simulink model "Four_Robots_v2"  (R2021a)
settings: Solver=FixedStepAuto  StartTime=0.0  StopTime=t_sim  FixedStep=0.01  RelTol=1e-3  EnableMultiTasking=on
model workspace (MAT data in the model file):
  SL_ROS_VariableLengthArrays_MaxSizes.CommonInfo.ArrayTruncateAction = 'EmitWarning'
  SL_ROS_VariableLengthArrays_MaxSizes.MsgTypeMap = containers.Map
  SL_ROS_VariableLengthArrays_MaxSizes.MsgTypeMap.serialization.keys = {'sensor_msgs/LaserScan'}
  SL_ROS_VariableLengthArrays_MaxSizes.MsgTypeMap.serialization.values{1}(1).PropertyName = 'Intensities'
  SL_ROS_VariableLengthArrays_MaxSizes.MsgTypeMap.serialization.values{1}(1).DataType = 'single'
  SL_ROS_VariableLengthArrays_MaxSizes.MsgTypeMap.serialization.values{1}(1).MaxLength = 360
  SL_ROS_VariableLengthArrays_MaxSizes.MsgTypeMap.serialization.values{1}(2).PropertyName = 'Ranges'
  SL_ROS_VariableLengthArrays_MaxSizes.MsgTypeMap.serialization.values{1}(2).DataType = 'single'
  SL_ROS_VariableLengthArrays_MaxSizes.MsgTypeMap.serialization.values{1}(2).MaxLength = 360
  SL_ROS_VariableLengthArrays_MaxSizes.MsgTypeMap.serialization.uniformity = 0
  SL_ROS_VariableLengthArrays_MaxSizes.MsgTypeMap.serialization.keyType = 'char'
  SL_ROS_VariableLengthArrays_MaxSizes.MsgTypeMap.serialization.valueType = 'any'
undefined symbols (not defined in the file or in its folder): Angular, Linear, PP, Way1, Way2, Way3, Way4
libraries: robotlib x16, robotalgslib x8
(part 1 of 2)
settings Model: EnablePacing=on  PacingRate=0.500000  Creator=The MathWorks, Inc.  LastModifiedBy=marco
settings SolverCC: AlgebraicLoopSolver=TrustRegion
settings DataIOCC: ReturnWorkspaceOutputs=off
settings OptimizationCC: EnhancedBackFolding=on  PassReuseOutputArgsAs=Individual arguments  ZeroExternalMemoryAtStartup=off  ZeroInternalMemoryAtStartup=off  MaxStackSize=64  OptimizeBlockOrder=speed  DifferentSizesBufferReuse=on  OptimizationCustomize=off  EfficientTunableParamExpr=on
settings DebuggingCC: ParameterTunabilityLossMsg=error  SFMachineParentedDataDiag=warning  ArithmeticOperatorsInVariantConditions=warning
settings HardwareCC: ProdBitPerPointer=32  ProdBitPerSizeT=32  ProdBitPerPtrDiffT=32  ProdLargestAtomicFloat=None  ProdIntDivRoundTo=Undefined  ProdEndianess=Unspecified  ProdWordSize=32  ProdHWDeviceType=Generic->Unspecified (assume 32-bit Generic)  UseEmbeddedCoderFeatures=off
settings SFSimCC: SimUseLocalCustomCode=off  MATLABDynamicMemAlloc=off  CustomCodeUndefinedFunction=UseInterfaceOnly
settings RTWCC: SystemTargetFile=ert.tlc  HardwareBoard=Robot Operating System (ROS)  TLCOptions="-aInlineSetEventsForThisBaseRateFcn=TLC_FALSE -aSuppressMultiTaskScheduler=TLC_FALSE  -aRateBasedStepFcn=0"  TemplateMakefile=ert_default_tmf  RTWUseLocalCustomCode=off  Toolchain=Catkin  TargetLang=C++
settings CodeAppCC: ForceParamTrailComments=on  IgnoreCustomStorageClasses=off  OperatorAnnotations=on  SimulinkDataObjDesc=on  SFDataObjDesc=on  InsertBlockDesc=on
settings ERTTargetCC: SupportNonInlinedSFcns=on
settings ConfigComp: CovMetricSettings=dsw  CovSaveCumulativeToWorkspaceVar=on  CovSaveSingleToWorkspaceVar=on  CovExternalEMLEnable=off

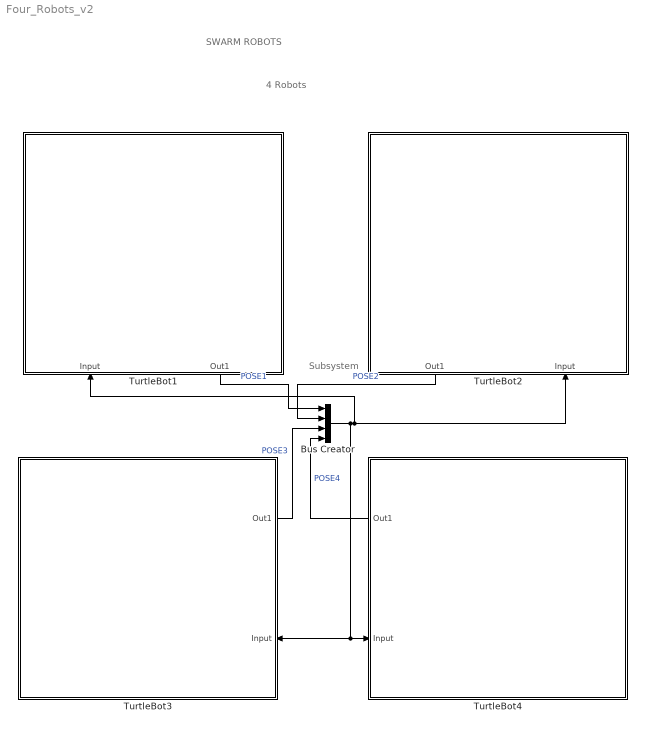
== system Four_Robots_v2 ==
  note: Subsystem
  note: SWARM ROBOTS
  note: 4 Robots
  Bus Creator : BusCreator  Inputs=4
  TurtleBot1 : Subsystem
      settings: PortSchema="{\"entries\":[{\"content\":{\"sides\":[{\"content\":{\"connectorIds\":[]},\"type\":\"ConnectorPlacement.EquallySpacedRectSide\",\"uuid\":\"56c3e334-5ee0-4d0f-bf2d-e3f55ae76ba4\"},{\"content\":{\"connectorIds\":[],\"side\":\"RIGHT\"},\"type\":\"ConnectorPlacement.EquallySpacedRectSide\",\"uuid\":\"47758117-cc89-48fb-b706-08d6cc9894c6\"},{\"content\":{\"connectorIds\":[],\"side\":\"TOP\"},\"type\":\"ConnectorPlacement.EquallySpacedRectSide\",\"uuid\":\"32d58290-5d9c-4684-a8aa-f76b0bdbcb35\"},{\"content\":{\"connectorIds\":[\"In1\",\"Out1\"],\"side\":\"BOTTOM\"},\"type\":\"ConnectorPlacement.EquallySpacedRectSide\",\"uuid\":\"a9083434-cc76-40d6-8718-10f7a0d9809f\"}]},\"type\":\"ConnectorPlacement.EquallySpacedConnector\",\"uuid\":\"5600436c-2c80-47b5-8769-67b5c2349f50\"}],\"packageUris\":[\"http://schema.mathworks.com/mf0/Connector/R2020b\"],\"version\":\"1.0\"}"
      mask Display: image('$imagefile'); % Use "Edit Image" on toolstrip to change.
  TurtleBot2 : Subsystem
      settings: PortSchema="{\"entries\":[{\"content\":{\"sides\":[{\"content\":{\"connectorIds\":[]},\"type\":\"ConnectorPlacement.EquallySpacedRectSide\",\"uuid\":\"56c3e334-5ee0-4d0f-bf2d-e3f55ae76ba4\"},{\"content\":{\"connectorIds\":[],\"side\":\"RIGHT\"},\"type\":\"ConnectorPlacement.EquallySpacedRectSide\",\"uuid\":\"47758117-cc89-48fb-b706-08d6cc9894c6\"},{\"content\":{\"connectorIds\":[],\"side\":\"TOP\"},\"type\":\"ConnectorPlacement.EquallySpacedRectSide\",\"uuid\":\"32d58290-5d9c-4684-a8aa-f76b0bdbcb35\"},{\"content\":{\"connectorIds\":[\"Out1\",\"In1\"],\"side\":\"BOTTOM\"},\"type\":\"ConnectorPlacement.EquallySpacedRectSide\",\"uuid\":\"a64cd998-99c6-4a68-9341-9505ecc52048\"}]},\"type\":\"ConnectorPlacement.EquallySpacedConnector\",\"uuid\":\"5600436c-2c80-47b5-8769-67b5c2349f50\"}],\"packageUris\":[\"http://schema.mathworks.com/mf0/Connector/R2020b\"],\"version\":\"1.0\"}"
      mask Display: image('$imagefile'); % Use "Edit Image" on toolstrip to change.
  TurtleBot3 : Subsystem
      settings: PortSchema="{\"entries\":[{\"content\":{\"sides\":[{\"content\":{\"connectorIds\":[]},\"type\":\"ConnectorPlacement.EquallySpacedRectSide\",\"uuid\":\"56c3e334-5ee0-4d0f-bf2d-e3f55ae76ba4\"},{\"content\":{\"connectorIds\":[\"Out1\",\"In1\"],\"side\":\"RIGHT\"},\"type\":\"ConnectorPlacement.EquallySpacedRectSide\",\"uuid\":\"47758117-cc89-48fb-b706-08d6cc9894c6\"},{\"content\":{\"connectorIds\":[],\"side\":\"TOP\"},\"type\":\"ConnectorPlacement.EquallySpacedRectSide\",\"uuid\":\"32d58290-5d9c-4684-a8aa-f76b0bdbcb35\"}]},\"type\":\"ConnectorPlacement.EquallySpacedConnector\",\"uuid\":\"5600436c-2c80-47b5-8769-67b5c2349f50\"}],\"packageUris\":[\"http://schema.mathworks.com/mf0/Connector/R2020b\"],\"version\":\"1.0\"}"
      mask Display: image('$imagefile'); % Use "Edit Image" on toolstrip to change.
  TurtleBot4 : Subsystem
      settings: PortSchema="{\"entries\":[{\"content\":{\"sides\":[{\"content\":{\"connectorIds\":[\"Out1\",\"In1\"]},\"type\":\"ConnectorPlacement.EquallySpacedRectSide\",\"uuid\":\"329d0968-fe7b-48af-96d4-efcc8444baaa\"},{\"content\":{\"connectorIds\":[],\"side\":\"RIGHT\"},\"type\":\"ConnectorPlacement.EquallySpacedRectSide\",\"uuid\":\"6b63acff-04c0-4cf0-89c5-b9cc2038ae37\"},{\"content\":{\"connectorIds\":[],\"side\":\"TOP\"},\"type\":\"ConnectorPlacement.EquallySpacedRectSide\",\"uuid\":\"86dad342-95f2-4c72-a91f-a7852aa38f6d\"}]},\"type\":\"ConnectorPlacement.EquallySpacedConnector\",\"uuid\":\"8a373283-c962-469e-9517-5e5763347250\"}],\"packageUris\":[\"http://schema.mathworks.com/mf0/Connector/R2020b\"],\"version\":\"1.0\"}"
      mask Display: image('$imagefile'); % Use "Edit Image" on toolstrip to change.
  wires:
  Bus Creator/1 -> TurtleBot4/1(Input), TurtleBot3/1(Input), TurtleBot1/1(Input), TurtleBot2/1(Input)
  TurtleBot3/1(Out1) -> Bus Creator/3  "POSE3"
  TurtleBot2/1(Out1) -> Bus Creator/2  "POSE2"
  TurtleBot4/1(Out1) -> Bus Creator/4  "POSE4"
  TurtleBot1/1(Out1) -> Bus Creator/1  "POSE1"

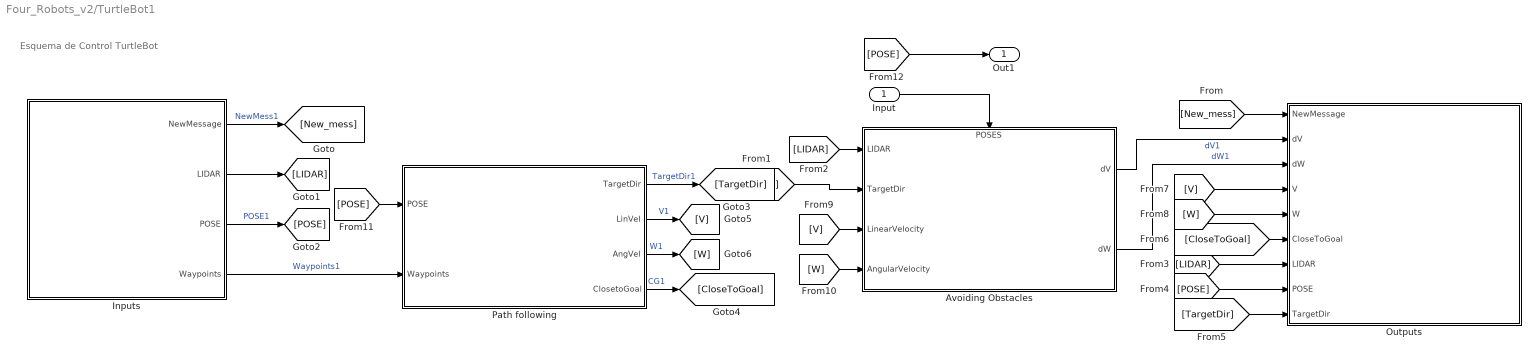
== system Four_Robots_v2/TurtleBot1 ==
  note: Esquema de Control TurtleBot
  Input : Inport
  " Avoiding Obstacles" : Subsystem
      settings: PortSchema="{\"entries\":[{\"content\":{\"sides\":[{\"content\":{\"connectorIds\":[\"In1\",\"In2\",\"In3\",\"In4\"]},\"type\":\"ConnectorPlacement.EquallySpacedRectSide\",\"uuid\":\"727160c1-1339-4bf3-a065-3e6cd81c52df\"},{\"content\":{\"connectorIds\":[\"Out1\",\"Out2\"],\"side\":\"RIGHT\"},\"type\":\"ConnectorPlacement.EquallySpacedRectSide\",\"uuid\":\"5e522eed-56ec-44ed-85e8-de700c46da17\"},{\"content\":{\"connectorIds\":[\"In5\"],\"side\":\"TOP\"},\"type\":\"ConnectorPlacement.EquallySpacedRectSide\",\"uuid\":\"c128634c-8085-427a-ae3a-e5a428db6a0b\"}]},\"type\":\"ConnectorPlacement.EquallySpacedConnector\",\"uuid\":\"85c8e4f2-74e0-4ae3-8945-7ca4be034673\"}],\"packageUris\":[\"http://schema.mathworks.com/mf0/Connector/R2020b\"],\"version\":\"1.0\"}"
      mask Display: image('$imagefile'); % Use "Edit Image" on toolstrip to change.
  " Path following" : Subsystem
      mask Display: image('$imagefile'); % Use "Edit Image" on toolstrip to change.
  Inputs : Subsystem
      mask Display: image('$imagefile'); % Use "Edit Image" on toolstrip to change.
  Outputs : Subsystem
      mask Display: image('$imagefile'); % Use "Edit Image" on toolstrip to change.
  Out1 : Outport
  wires:
  Inputs/3(POSE) -> [POSE]  "POSE1"
  Inputs/1(NewMessage) -> [New_mess]  "NewMess1"
  Inputs/2(LIDAR) -> [LIDAR]
  Inputs/4(Waypoints) -> " Path following"/2(Waypoints)  "Waypoints1"
  " Path following"/4(ClosetoGoal) -> [CloseToGoal]  "CG1"
  [LIDAR] -> " Avoiding Obstacles"/1(LIDAR)
  [New_mess] -> Outputs/1(NewMessage)
  [V] -> Outputs/4(V)
  [W] -> Outputs/5(W)
  [CloseToGoal] -> Outputs/6(CloseToGoal)
  [LIDAR] -> Outputs/7(LIDAR)
  [POSE] -> Outputs/8(POSE)
  [TargetDir] -> Outputs/9(TargetDir)
  " Path following"/1(TargetDir) -> [TargetDir]  "TargetDir1"
  " Avoiding Obstacles"/1(dV) -> Outputs/2(dV)  "dV1"
  " Avoiding Obstacles"/2(dW) -> Outputs/3(dW)  "dW1"
  " Path following"/3(AngVel) -> [W]  "W1"
  " Path following"/2(LinVel) -> [V]  "V1"
  [TargetDir] -> " Avoiding Obstacles"/2(TargetDir)
  [V] -> " Avoiding Obstacles"/3(LinearVelocity)
  [W] -> " Avoiding Obstacles"/4(AngularVelocity)
  [POSE] -> " Path following"/1(POSE)
  [POSE] -> Out1/1
  Input/1 -> " Avoiding Obstacles"/5(POSES)

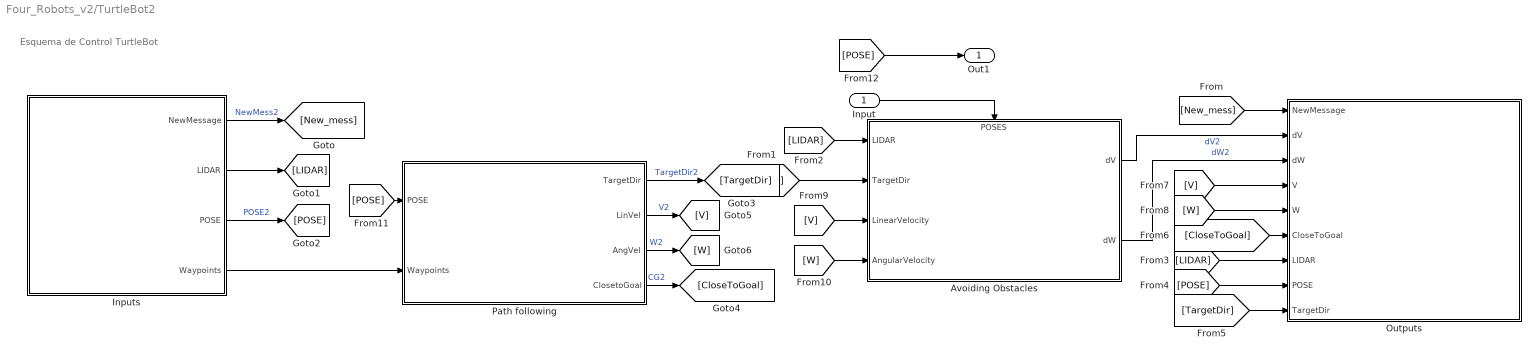
== system Four_Robots_v2/TurtleBot2 ==
  note: Esquema de Control TurtleBot
  Input : Inport
  " Avoiding Obstacles" : Subsystem
      settings: PortSchema="{\"entries\":[{\"content\":{\"sides\":[{\"content\":{\"connectorIds\":[\"In1\",\"In2\",\"In3\",\"In4\"]},\"type\":\"ConnectorPlacement.EquallySpacedRectSide\",\"uuid\":\"727160c1-1339-4bf3-a065-3e6cd81c52df\"},{\"content\":{\"connectorIds\":[\"Out1\",\"Out2\"],\"side\":\"RIGHT\"},\"type\":\"ConnectorPlacement.EquallySpacedRectSide\",\"uuid\":\"5e522eed-56ec-44ed-85e8-de700c46da17\"},{\"content\":{\"connectorIds\":[\"In5\"],\"side\":\"TOP\"},\"type\":\"ConnectorPlacement.EquallySpacedRectSide\",\"uuid\":\"c128634c-8085-427a-ae3a-e5a428db6a0b\"}]},\"type\":\"ConnectorPlacement.EquallySpacedConnector\",\"uuid\":\"85c8e4f2-74e0-4ae3-8945-7ca4be034673\"}],\"packageUris\":[\"http://schema.mathworks.com/mf0/Connector/R2020b\"],\"version\":\"1.0\"}"
      mask Display: image('$imagefile'); % Use "Edit Image" on toolstrip to change.
  " Path following" : Subsystem
      mask Display: image('$imagefile'); % Use "Edit Image" on toolstrip to change.
  Inputs : Subsystem
      mask Display: image('$imagefile'); % Use "Edit Image" on toolstrip to change.
  Outputs : Subsystem
      mask Display: image('$imagefile'); % Use "Edit Image" on toolstrip to change.
  Out1 : Outport
  wires:
  Inputs/3(POSE) -> [POSE]  "POSE2"
  Inputs/1(NewMessage) -> [New_mess]  "NewMess2"
  Inputs/2(LIDAR) -> [LIDAR]
  Inputs/4(Waypoints) -> " Path following"/2(Waypoints)
  " Path following"/4(ClosetoGoal) -> [CloseToGoal]  "CG2"
  [LIDAR] -> " Avoiding Obstacles"/1(LIDAR)
  [New_mess] -> Outputs/1(NewMessage)
  [V] -> Outputs/4(V)
  [W] -> Outputs/5(W)
  [CloseToGoal] -> Outputs/6(CloseToGoal)
  [LIDAR] -> Outputs/7(LIDAR)
  [POSE] -> Outputs/8(POSE)
  [TargetDir] -> Outputs/9(TargetDir)
  " Path following"/1(TargetDir) -> [TargetDir]  "TargetDir2"
  " Avoiding Obstacles"/1(dV) -> Outputs/2(dV)  "dV2"
  " Avoiding Obstacles"/2(dW) -> Outputs/3(dW)  "dW2"
  " Path following"/3(AngVel) -> [W]  "W2"
  " Path following"/2(LinVel) -> [V]  "V2"
  [TargetDir] -> " Avoiding Obstacles"/2(TargetDir)
  [V] -> " Avoiding Obstacles"/3(LinearVelocity)
  [W] -> " Avoiding Obstacles"/4(AngularVelocity)
  [POSE] -> " Path following"/1(POSE)
  Input/1 -> " Avoiding Obstacles"/5(POSES)
  [POSE] -> Out1/1

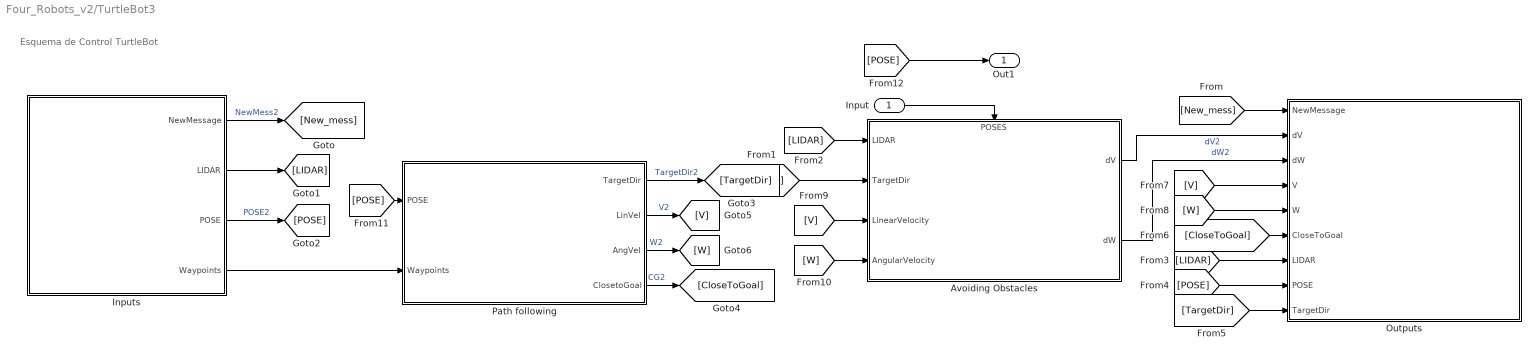
== system Four_Robots_v2/TurtleBot3 ==
  note: Esquema de Control TurtleBot
  Input : Inport
  " Avoiding Obstacles" : Subsystem
      settings: PortSchema="{\"entries\":[{\"content\":{\"sides\":[{\"content\":{\"connectorIds\":[\"In1\",\"In2\",\"In3\",\"In4\"]},\"type\":\"ConnectorPlacement.EquallySpacedRectSide\",\"uuid\":\"727160c1-1339-4bf3-a065-3e6cd81c52df\"},{\"content\":{\"connectorIds\":[\"Out1\",\"Out2\"],\"side\":\"RIGHT\"},\"type\":\"ConnectorPlacement.EquallySpacedRectSide\",\"uuid\":\"5e522eed-56ec-44ed-85e8-de700c46da17\"},{\"content\":{\"connectorIds\":[\"In5\"],\"side\":\"TOP\"},\"type\":\"ConnectorPlacement.EquallySpacedRectSide\",\"uuid\":\"c128634c-8085-427a-ae3a-e5a428db6a0b\"}]},\"type\":\"ConnectorPlacement.EquallySpacedConnector\",\"uuid\":\"85c8e4f2-74e0-4ae3-8945-7ca4be034673\"}],\"packageUris\":[\"http://schema.mathworks.com/mf0/Connector/R2020b\"],\"version\":\"1.0\"}"
      mask Display: image('$imagefile'); % Use "Edit Image" on toolstrip to change.
  " Path following" : Subsystem
      mask Display: image('$imagefile'); % Use "Edit Image" on toolstrip to change.
  Inputs : Subsystem
      mask Display: image('$imagefile'); % Use "Edit Image" on toolstrip to change.
  Outputs : Subsystem
      mask Display: image('$imagefile'); % Use "Edit Image" on toolstrip to change.
  Out1 : Outport
  wires:
  Inputs/3(POSE) -> [POSE]  "POSE2"
  Inputs/1(NewMessage) -> [New_mess]  "NewMess2"
  Inputs/2(LIDAR) -> [LIDAR]
  Inputs/4(Waypoints) -> " Path following"/2(Waypoints)
  " Path following"/4(ClosetoGoal) -> [CloseToGoal]  "CG2"
  [LIDAR] -> " Avoiding Obstacles"/1(LIDAR)
  [New_mess] -> Outputs/1(NewMessage)
  [V] -> Outputs/4(V)
  [W] -> Outputs/5(W)
  [CloseToGoal] -> Outputs/6(CloseToGoal)
  [LIDAR] -> Outputs/7(LIDAR)
  [POSE] -> Outputs/8(POSE)
  [TargetDir] -> Outputs/9(TargetDir)
  " Path following"/1(TargetDir) -> [TargetDir]  "TargetDir2"
  " Avoiding Obstacles"/1(dV) -> Outputs/2(dV)  "dV2"
  " Avoiding Obstacles"/2(dW) -> Outputs/3(dW)  "dW2"
  " Path following"/3(AngVel) -> [W]  "W2"
  " Path following"/2(LinVel) -> [V]  "V2"
  [TargetDir] -> " Avoiding Obstacles"/2(TargetDir)
  [V] -> " Avoiding Obstacles"/3(LinearVelocity)
  [W] -> " Avoiding Obstacles"/4(AngularVelocity)
  [POSE] -> " Path following"/1(POSE)
  [POSE] -> Out1/1
  Input/1 -> " Avoiding Obstacles"/5(POSES)

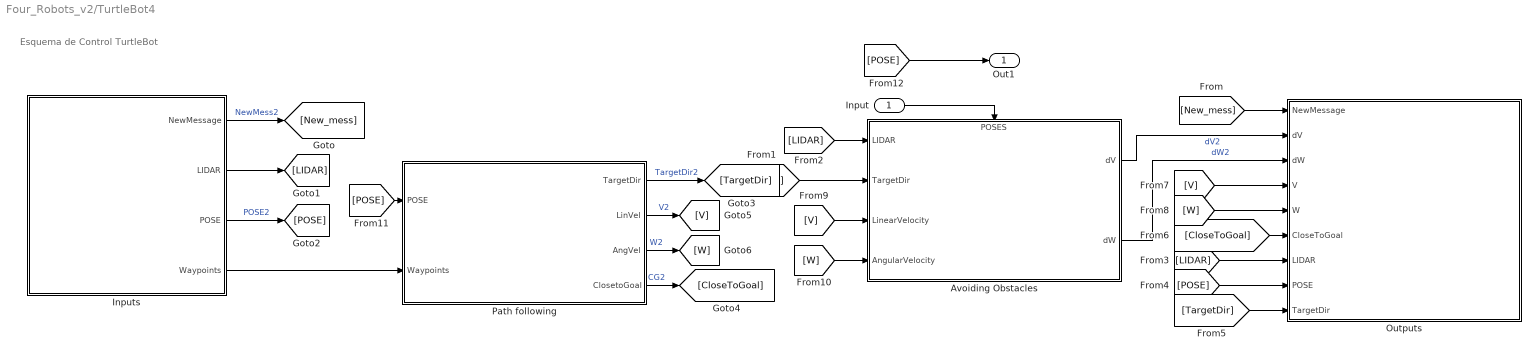
== system Four_Robots_v2/TurtleBot4 ==
  note: Esquema de Control TurtleBot
  Input : Inport
  " Avoiding Obstacles" : Subsystem
      settings: PortSchema="{\"entries\":[{\"content\":{\"sides\":[{\"content\":{\"connectorIds\":[\"In1\",\"In2\",\"In3\",\"In4\"]},\"type\":\"ConnectorPlacement.EquallySpacedRectSide\",\"uuid\":\"727160c1-1339-4bf3-a065-3e6cd81c52df\"},{\"content\":{\"connectorIds\":[\"Out1\",\"Out2\"],\"side\":\"RIGHT\"},\"type\":\"ConnectorPlacement.EquallySpacedRectSide\",\"uuid\":\"5e522eed-56ec-44ed-85e8-de700c46da17\"},{\"content\":{\"connectorIds\":[\"In5\"],\"side\":\"TOP\"},\"type\":\"ConnectorPlacement.EquallySpacedRectSide\",\"uuid\":\"c128634c-8085-427a-ae3a-e5a428db6a0b\"}]},\"type\":\"ConnectorPlacement.EquallySpacedConnector\",\"uuid\":\"85c8e4f2-74e0-4ae3-8945-7ca4be034673\"}],\"packageUris\":[\"http://schema.mathworks.com/mf0/Connector/R2020b\"],\"version\":\"1.0\"}"
      mask Display: image('$imagefile'); % Use "Edit Image" on toolstrip to change.
  " Path following" : Subsystem
      mask Display: image('$imagefile'); % Use "Edit Image" on toolstrip to change.
  Inputs : Subsystem
      mask Display: image('$imagefile'); % Use "Edit Image" on toolstrip to change.
  Outputs : Subsystem
      mask Display: image('$imagefile'); % Use "Edit Image" on toolstrip to change.
  Out1 : Outport
  wires:
  Input/1 -> " Avoiding Obstacles"/5(POSES)
  [POSE] -> Out1/1
  [POSE] -> " Path following"/1(POSE)
  [W] -> " Avoiding Obstacles"/4(AngularVelocity)
  [V] -> " Avoiding Obstacles"/3(LinearVelocity)
  [TargetDir] -> " Avoiding Obstacles"/2(TargetDir)
  " Path following"/2(LinVel) -> [V]  "V2"
  " Path following"/3(AngVel) -> [W]  "W2"
  " Avoiding Obstacles"/2(dW) -> Outputs/3(dW)  "dW2"
  " Avoiding Obstacles"/1(dV) -> Outputs/2(dV)  "dV2"
  " Path following"/1(TargetDir) -> [TargetDir]  "TargetDir2"
  [TargetDir] -> Outputs/9(TargetDir)
  [POSE] -> Outputs/8(POSE)
  [LIDAR] -> Outputs/7(LIDAR)
  [CloseToGoal] -> Outputs/6(CloseToGoal)
  [W] -> Outputs/5(W)
  [V] -> Outputs/4(V)
  [New_mess] -> Outputs/1(NewMessage)
  [LIDAR] -> " Avoiding Obstacles"/1(LIDAR)
  " Path following"/4(ClosetoGoal) -> [CloseToGoal]  "CG2"
  Inputs/4(Waypoints) -> " Path following"/2(Waypoints)
  Inputs/2(LIDAR) -> [LIDAR]
  Inputs/1(NewMessage) -> [New_mess]  "NewMess2"
  Inputs/3(POSE) -> [POSE]  "POSE2"

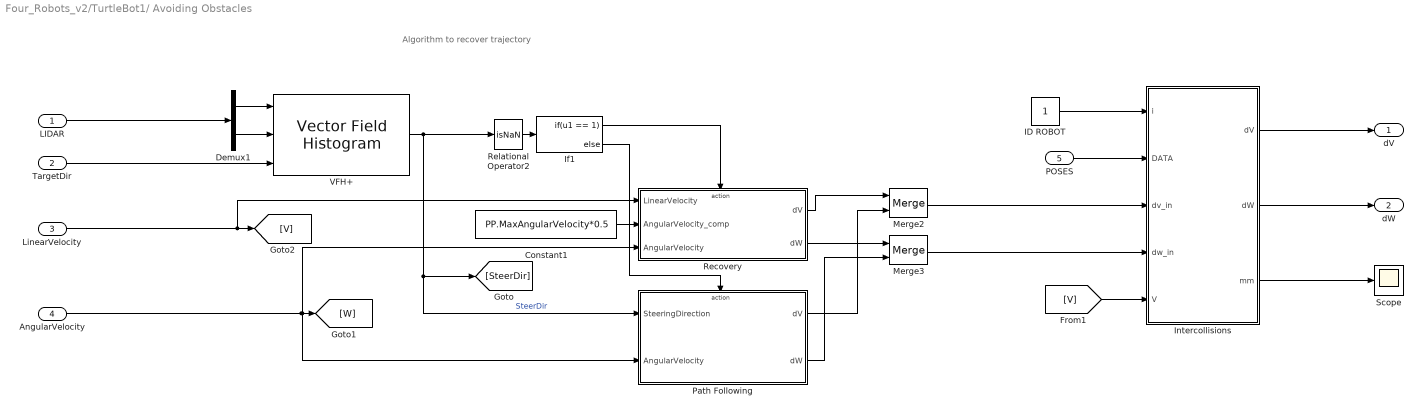
== system Four_Robots_v2/TurtleBot1/ Avoiding Obstacles ==
  note: Algorithm to recover trajectory
  LIDAR : Inport
  TargetDir : Inport  Port=2
  LinearVelocity : Inport  Port=3
  AngularVelocity : Inport  Port=4
  POSES : Inport  Port=5
  Constant1 : Constant  Value=PP.MaxAngularVelocity*0.5
  Demux1 : Demux  Outputs=2
  ID ROBOT : Constant
  If1 : If  IfExpression=u1 == 1
  Intercollisions : MATLAB Function  TreatAsAtomicUnit=on
  Merge2 : Merge
  Merge3 : Merge
  Path Following : Subsystem  TreatAsAtomicUnit=on
  Recovery : Subsystem  TreatAsAtomicUnit=on
  Relational Operator2 : RelationalOperator  Operator=isNaN  OutDataTypeStr=boolean  RndMeth=Simplest
  Scope : Scope
  VFH+ : robotalgslib/Vector Field Histogram  NumAngularSectors=VFH.NumAngularSectors  DistanceLimits=VFH.DistanceLimits  HistogramThresholds=VFH.HistogramThresholds  RobotRadius=VFH.RobotRadius  SafetyDistance=VFH.SafetyDistance  MinTurningRadius=VFH.MinTurningRadius  SimulateUsing=Code generation  TargetDirectionWeight=5  CurrentDirectionWeight=2  PreviousDirectionWeight=2
      settings: SourceProductBaseCode=NV,RO
  dV : Outport
  dW : Outport  Port=2
  wires:
  If1/1 -> Recovery/Action
  Constant1/1 -> Recovery/2(AngularVelocity_comp)
  Recovery/1(dV) -> Merge2/1
  Recovery/2(dW) -> Merge3/1
  AngularVelocity/1 -> Recovery/3(AngularVelocity), Path Following/2(AngularVelocity), [W]
  Demux1/1 -> VFH+/1
  TargetDir/1 -> VFH+/3
  Relational Operator2/1 -> If1/1
  LinearVelocity/1 -> [V], Recovery/1(LinearVelocity)
  LIDAR/1 -> Demux1/1
  VFH+/1 -> [SteerDir], Path Following/1(SteeringDirection), Relational Operator2/1  "SteerDir"
  Path Following/2(dW) -> Merge3/2
  Path Following/1(dV) -> Merge2/2
  If1/2 -> Path Following/Action
  Demux1/2 -> VFH+/2
  Intercollisions/2(dW) -> dW/1
  [V] -> Intercollisions/5(V)
  Merge2/1 -> Intercollisions/3(dv_in)
  Merge3/1 -> Intercollisions/4(dw_in)
  Intercollisions/1(dV) -> dV/1
  ID ROBOT/1 -> Intercollisions/1(i)
  POSES/1 -> Intercollisions/2(DATA)
  Intercollisions/3(mm) -> Scope/1

== system Four_Robots_v2/TurtleBot1/ Path following ==
  note: Check If Close To Goal
  POSE : Inport
  Waypoints : Inport  Port=2
  " Extract Goal" : MATLAB Function  TreatAsAtomicUnit=on
  Dot Product : DotProduct  InputSameDT=on  OutDataTypeStr=Inherit: Inherit via internal rule
  GoalRadius : Constant  Value=0.15
  Pure Pursuit : robotalgslib/Pure Pursuit  DesiredLinearVelocity=PP.DesiredLinearVelocity  MaxAngularVelocity=PP.MaxAngularVelocity  LookaheadDistance=PP.LookaheadDistance  TargetDirPort=on  SimulateUsing=Code generation
  Relational Operator : RelationalOperator  Operator=<=  OutDataTypeStr=boolean  RndMeth=Simplest
  Selector : Selector  InputPortWidth=3  IndexOptions=Index vector (dialog)  Indices=[1 2]  OutputSizes=1
  Sqrt : Sqrt  SaturateOnIntegerOverflow=on
  Subtract : Sum  Inputs=|+-
  TargetDir : Outport
  LinVel : Outport  Port=2
  AngVel : Outport  Port=3
  ClosetoGoal : Outport  Port=4
  wires:
  Pure Pursuit/3 -> TargetDir/1
  Pure Pursuit/2 -> AngVel/1
  Relational Operator/1 -> ClosetoGoal/1
  Subtract/1 -> Dot Product/1, Dot Product/2
  " Extract Goal"/1(Goal) -> Subtract/2
  Dot Product/1 -> Sqrt/1
  Pure Pursuit/1 -> LinVel/1
  Selector/1 -> Subtract/1
  Waypoints/1 -> " Extract Goal"/1(Waypoints), Pure Pursuit/2
  Sqrt/1 -> Relational Operator/1
  GoalRadius/1 -> Relational Operator/2
  POSE/1 -> Selector/1, Pure Pursuit/1

== system Four_Robots_v2/TurtleBot1/Inputs ==
  note: Receive Laser Message
  note: Receive Robot Pose
  Bus Selector : BusSelector  OutputSignals=Pose.Pose.Position.X,Pose.Pose.Position.Y,Pose.Pose.Orientation.X,Pose.Pose.Orientation.Y,Pose.Pose.Orientation.Z,Pose.Pose.Orientation.W
  MATLAB Function : MATLAB Function  TreatAsAtomicUnit=on
  Mux : Mux  Inputs=3
  Mux1 : Mux  Inputs=2
  Subscribe : robotlib/Subscribe  topicSource=Select from ROS network  topic=/robot1/scan  messageType=sensor_msgs/LaserScan  SampleTime=-1  legacyBusStruct=off  messageQueueLength=1
  Subscribe1 : robotlib/Subscribe  topicSource=Select from ROS network  topic=/robot1/odom  messageType=nav_msgs/Odometry  SampleTime=-1  legacyBusStruct=off  messageQueueLength=1
  Terminator : Terminator
  Waypoints Input1 : Constant  Value=Way1  OutDataTypeStr=double
  quad2eul : MATLAB Function  TreatAsAtomicUnit=on
  NewMessage : Outport
  LIDAR : Outport  Port=2
  POSE : Outport  Port=3
  Waypoints : Outport  Port=4
  wires:
  Bus Selector/6 -> quad2eul/4(W)  "<W>"
  Bus Selector/1 -> Mux/1  "<X>"
  quad2eul/1(Yaw) -> Mux/3
  Bus Selector/4 -> quad2eul/2(Y)  "<Y>"
  Subscribe1/2 -> Bus Selector/1
  MATLAB Function/1(Ranges) -> Mux1/1
  Mux/1 -> POSE/1
  Subscribe/2 -> MATLAB Function/1(LaserScanMsg)
  Subscribe/1 -> NewMessage/1
  Subscribe1/1 -> Terminator/1
  Bus Selector/3 -> quad2eul/1(X)  "<X>"
  Bus Selector/2 -> Mux/2  "<Y>"
  MATLAB Function/2(Angles) -> Mux1/2
  Mux1/1 -> LIDAR/1
  Waypoints Input1/1 -> Waypoints/1
  Bus Selector/5 -> quad2eul/3(Z)  "<Z>"

== system Four_Robots_v2/TurtleBot1/Outputs ==
  NewMessage : Inport
  dV : Inport  Port=2
  dW : Inport  Port=3
  V : Inport  Port=4
  W : Inport  Port=5
  CloseToGoal : Inport  Port=6
  LIDAR : Inport  Port=7
  POSE : Inport  Port=8
  TargetDir : Inport  Port=9
  DVelocities : Scope  NumInputPorts=2
  Outputs : Subsystem
  wires:
  POSE/1 -> Outputs/7(POSE)
  V/1 -> Outputs/3(V)
  NewMessage/1 -> Outputs/Enable
  CloseToGoal/1 -> Outputs/5(CloseToGoal)
  LIDAR/1 -> Outputs/6(LIDAR)
  TargetDir/1 -> Outputs/8(TargetDir)
  W/1 -> Outputs/4(W)
  dV/1 -> DVelocities/1, Outputs/1(dV)
  dW/1 -> DVelocities/2, Outputs/2(dW)

== system Four_Robots_v2/TurtleBot2/ Avoiding Obstacles ==
  note: Algorithm to recover trajectory
  LIDAR : Inport
  TargetDir : Inport  Port=2
  LinearVelocity : Inport  Port=3
  AngularVelocity : Inport  Port=4
  POSES : Inport  Port=5
  Constant1 : Constant  Value=PP.MaxAngularVelocity*0.5
  Demux1 : Demux  Outputs=2
  ID ROBOT : Constant  Value=2
  If1 : If  IfExpression=u1 == 1
  Intercollisions : MATLAB Function  TreatAsAtomicUnit=on
  Merge2 : Merge
  Merge3 : Merge
  Path Following : Subsystem  TreatAsAtomicUnit=on
  Recovery : Subsystem  TreatAsAtomicUnit=on
  Relational Operator2 : RelationalOperator  Operator=isNaN  OutDataTypeStr=boolean  RndMeth=Simplest
  VFH+ : robotalgslib/Vector Field Histogram  NumAngularSectors=VFH.NumAngularSectors  DistanceLimits=VFH.DistanceLimits  HistogramThresholds=VFH.HistogramThresholds  RobotRadius=VFH.RobotRadius  SafetyDistance=VFH.SafetyDistance  MinTurningRadius=VFH.MinTurningRadius  SimulateUsing=Code generation  TargetDirectionWeight=5  CurrentDirectionWeight=2  PreviousDirectionWeight=2
      settings: SourceProductBaseCode=NV,RO
  dV : Outport
  dW : Outport  Port=2
  wires:
  If1/1 -> Recovery/Action
  Constant1/1 -> Recovery/2(AngularVelocity_comp)
  Recovery/1(dV) -> Merge2/1
  Recovery/2(dW) -> Merge3/1
  AngularVelocity/1 -> Recovery/3(AngularVelocity), Path Following/2(AngularVelocity), [W]
  Demux1/1 -> VFH+/1
  TargetDir/1 -> VFH+/3
  Relational Operator2/1 -> If1/1
  LinearVelocity/1 -> [V], Recovery/1(LinearVelocity)
  LIDAR/1 -> Demux1/1
  VFH+/1 -> [SteerDir], Path Following/1(SteeringDirection), Relational Operator2/1  "SteerDir"
  Path Following/2(dW) -> Merge3/2
  Path Following/1(dV) -> Merge2/2
  If1/2 -> Path Following/Action
  Demux1/2 -> VFH+/2
  Intercollisions/2(dW) -> dW/1
  ID ROBOT/1 -> Intercollisions/1(i)
  POSES/1 -> Intercollisions/2(DATA)
  Merge2/1 -> Intercollisions/3(dv_in)
  [V] -> Intercollisions/5(V)
  Merge3/1 -> Intercollisions/4(dw_in)
  Intercollisions/1(dV) -> dV/1

== system Four_Robots_v2/TurtleBot2/ Path following ==
  note: Check If Close To Goal
  POSE : Inport
  Waypoints : Inport  Port=2
  " Extract Goal" : MATLAB Function  TreatAsAtomicUnit=on
  Dot Product : DotProduct  InputSameDT=on  OutDataTypeStr=Inherit: Inherit via internal rule
  GoalRadius : Constant  Value=0.15
  Pure Pursuit : robotalgslib/Pure Pursuit  DesiredLinearVelocity=PP.DesiredLinearVelocity  MaxAngularVelocity=PP.MaxAngularVelocity  LookaheadDistance=PP.LookaheadDistance  TargetDirPort=on  SimulateUsing=Code generation
  Relational Operator : RelationalOperator  Operator=<=  OutDataTypeStr=boolean  RndMeth=Simplest
  Selector : Selector  InputPortWidth=3  IndexOptions=Index vector (dialog)  Indices=[1 2]  OutputSizes=1
  Sqrt : Sqrt  SaturateOnIntegerOverflow=on
  Subtract : Sum  Inputs=|+-
  TargetDir : Outport
  LinVel : Outport  Port=2
  AngVel : Outport  Port=3
  ClosetoGoal : Outport  Port=4
  wires:
  Pure Pursuit/3 -> TargetDir/1
  Pure Pursuit/2 -> AngVel/1
  Relational Operator/1 -> ClosetoGoal/1
  Subtract/1 -> Dot Product/1, Dot Product/2
  " Extract Goal"/1(Goal) -> Subtract/2
  Dot Product/1 -> Sqrt/1
  Pure Pursuit/1 -> LinVel/1
  Selector/1 -> Subtract/1
  Waypoints/1 -> " Extract Goal"/1(Waypoints), Pure Pursuit/2
  Sqrt/1 -> Relational Operator/1
  GoalRadius/1 -> Relational Operator/2
  POSE/1 -> Selector/1, Pure Pursuit/1

== system Four_Robots_v2/TurtleBot2/Inputs ==
  note: Receive Laser Message
  note: Receive Robot Pose
  Bus Selector : BusSelector  OutputSignals=Pose.Pose.Position.X,Pose.Pose.Position.Y,Pose.Pose.Orientation.X,Pose.Pose.Orientation.Y,Pose.Pose.Orientation.Z,Pose.Pose.Orientation.W
  MATLAB Function : MATLAB Function  TreatAsAtomicUnit=on
  Mux : Mux  Inputs=3
  Mux1 : Mux  Inputs=2
  Subscribe : robotlib/Subscribe  topicSource=Select from ROS network  topic=/robot2/scan  messageType=sensor_msgs/LaserScan  SampleTime=-1  legacyBusStruct=off  messageQueueLength=1
  Subscribe1 : robotlib/Subscribe  topicSource=Select from ROS network  topic=/robot2/odom  messageType=nav_msgs/Odometry  SampleTime=-1  legacyBusStruct=off  messageQueueLength=1
  Terminator : Terminator
  Waypoints Input1 : Constant  Value=Way2  OutDataTypeStr=double
  quad2eul : MATLAB Function  TreatAsAtomicUnit=on
  NewMessage : Outport
  LIDAR : Outport  Port=2
  POSE : Outport  Port=3
  Waypoints : Outport  Port=4
  wires:
  Bus Selector/6 -> quad2eul/4(W)  "<W>"
  Bus Selector/1 -> Mux/1  "<X>"
  quad2eul/1(Yaw) -> Mux/3
  Bus Selector/4 -> quad2eul/2(Y)  "<Y>"
  Subscribe1/2 -> Bus Selector/1
  MATLAB Function/1(Ranges) -> Mux1/1
  Mux/1 -> POSE/1
  Subscribe/2 -> MATLAB Function/1(LaserScanMsg)
  Subscribe/1 -> NewMessage/1
  Subscribe1/1 -> Terminator/1
  Bus Selector/3 -> quad2eul/1(X)  "<X>"
  Bus Selector/2 -> Mux/2  "<Y>"
  MATLAB Function/2(Angles) -> Mux1/2
  Mux1/1 -> LIDAR/1
  Waypoints Input1/1 -> Waypoints/1
  Bus Selector/5 -> quad2eul/3(Z)  "<Z>"

== system Four_Robots_v2/TurtleBot2/Outputs ==
  NewMessage : Inport
  dV : Inport  Port=2
  dW : Inport  Port=3
  V : Inport  Port=4
  W : Inport  Port=5
  CloseToGoal : Inport  Port=6
  LIDAR : Inport  Port=7
  POSE : Inport  Port=8
  TargetDir : Inport  Port=9
  DVelocities : Scope  NumInputPorts=2
  Outputs : Subsystem
  wires:
  POSE/1 -> Outputs/7(POSE)
  V/1 -> Outputs/3(V)
  NewMessage/1 -> Outputs/Enable
  CloseToGoal/1 -> Outputs/5(CloseToGoal)
  LIDAR/1 -> Outputs/6(LIDAR)
  TargetDir/1 -> Outputs/8(TargetDir)
  W/1 -> Outputs/4(W)
  dV/1 -> DVelocities/1, Outputs/1(dV)
  dW/1 -> DVelocities/2, Outputs/2(dW)

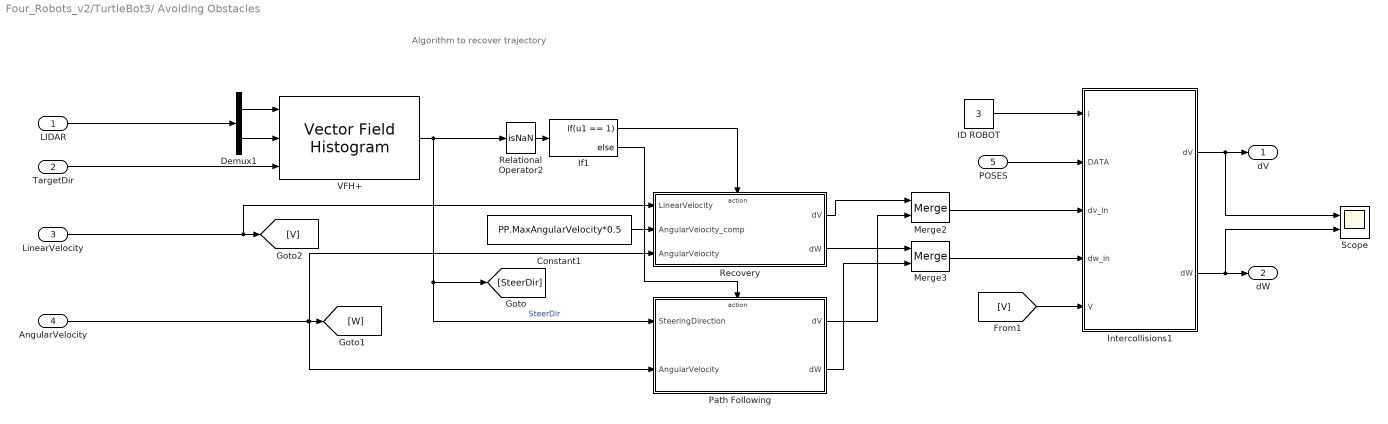
== system Four_Robots_v2/TurtleBot3/ Avoiding Obstacles ==
  note: Algorithm to recover trajectory
  LIDAR : Inport
  TargetDir : Inport  Port=2
  LinearVelocity : Inport  Port=3
  AngularVelocity : Inport  Port=4
  POSES : Inport  Port=5
  Constant1 : Constant  Value=PP.MaxAngularVelocity*0.5
  Demux1 : Demux  Outputs=2
  ID ROBOT : Constant  Value=3
  If1 : If  IfExpression=u1 == 1
  Intercollisions1 : MATLAB Function  TreatAsAtomicUnit=on
  Merge2 : Merge
  Merge3 : Merge
  Path Following : Subsystem  TreatAsAtomicUnit=on
  Recovery : Subsystem  TreatAsAtomicUnit=on
  Relational Operator2 : RelationalOperator  Operator=isNaN  OutDataTypeStr=boolean  RndMeth=Simplest
  Scope : Scope  NumInputPorts=2
  VFH+ : robotalgslib/Vector Field Histogram  NumAngularSectors=VFH.NumAngularSectors  DistanceLimits=VFH.DistanceLimits  HistogramThresholds=VFH.HistogramThresholds  RobotRadius=VFH.RobotRadius  SafetyDistance=VFH.SafetyDistance  MinTurningRadius=VFH.MinTurningRadius  SimulateUsing=Code generation  TargetDirectionWeight=5  CurrentDirectionWeight=2  PreviousDirectionWeight=2
      settings: SourceProductBaseCode=NV,RO
  dV : Outport
  dW : Outport  Port=2
  wires:
  If1/1 -> Recovery/Action
  Constant1/1 -> Recovery/2(AngularVelocity_comp)
  Recovery/1(dV) -> Merge2/1
  Recovery/2(dW) -> Merge3/1
  AngularVelocity/1 -> Recovery/3(AngularVelocity), Path Following/2(AngularVelocity), [W]
  Demux1/1 -> VFH+/1
  TargetDir/1 -> VFH+/3
  Relational Operator2/1 -> If1/1
  LinearVelocity/1 -> [V], Recovery/1(LinearVelocity)
  LIDAR/1 -> Demux1/1
  VFH+/1 -> [SteerDir], Path Following/1(SteeringDirection), Relational Operator2/1  "SteerDir"
  Path Following/2(dW) -> Merge3/2
  Path Following/1(dV) -> Merge2/2
  If1/2 -> Path Following/Action
  Demux1/2 -> VFH+/2
  Merge3/1 -> Intercollisions1/4(dw_in)
  [V] -> Intercollisions1/5(V)
  Merge2/1 -> Intercollisions1/3(dv_in)
  Intercollisions1/2(dW) -> Scope/2, dW/1
  Intercollisions1/1(dV) -> Scope/1, dV/1
  POSES/1 -> Intercollisions1/2(DATA)
  ID ROBOT/1 -> Intercollisions1/1(i)

== system Four_Robots_v2/TurtleBot3/ Path following ==
  note: Check If Close To Goal
  POSE : Inport
  Waypoints : Inport  Port=2
  " Extract Goal" : MATLAB Function  TreatAsAtomicUnit=on
  Dot Product : DotProduct  InputSameDT=on  OutDataTypeStr=Inherit: Inherit via internal rule
  GoalRadius : Constant  Value=0.15
  Pure Pursuit : robotalgslib/Pure Pursuit  DesiredLinearVelocity=PP.DesiredLinearVelocity  MaxAngularVelocity=PP.MaxAngularVelocity  LookaheadDistance=PP.LookaheadDistance  TargetDirPort=on  SimulateUsing=Code generation
  Relational Operator : RelationalOperator  Operator=<=  OutDataTypeStr=boolean  RndMeth=Simplest
  Selector : Selector  InputPortWidth=3  IndexOptions=Index vector (dialog)  Indices=[1 2]  OutputSizes=1
  Sqrt : Sqrt  SaturateOnIntegerOverflow=on
  Subtract : Sum  Inputs=|+-
  TargetDir : Outport
  LinVel : Outport  Port=2
  AngVel : Outport  Port=3
  ClosetoGoal : Outport  Port=4
  wires:
  Pure Pursuit/3 -> TargetDir/1
  Pure Pursuit/2 -> AngVel/1
  Relational Operator/1 -> ClosetoGoal/1
  Subtract/1 -> Dot Product/1, Dot Product/2
  " Extract Goal"/1(Goal) -> Subtract/2
  Dot Product/1 -> Sqrt/1
  Pure Pursuit/1 -> LinVel/1
  Selector/1 -> Subtract/1
  Waypoints/1 -> " Extract Goal"/1(Waypoints), Pure Pursuit/2
  Sqrt/1 -> Relational Operator/1
  GoalRadius/1 -> Relational Operator/2
  POSE/1 -> Selector/1, Pure Pursuit/1

== system Four_Robots_v2/TurtleBot3/Inputs ==
  note: Receive Laser Message
  note: Receive Robot Pose
  Bus Selector : BusSelector  OutputSignals=Pose.Pose.Position.X,Pose.Pose.Position.Y,Pose.Pose.Orientation.X,Pose.Pose.Orientation.Y,Pose.Pose.Orientation.Z,Pose.Pose.Orientation.W
  MATLAB Function : MATLAB Function  TreatAsAtomicUnit=on
  Mux : Mux  Inputs=3
  Mux1 : Mux  Inputs=2
  Subscribe : robotlib/Subscribe  topicSource=Select from ROS network  topic=/robot3/scan  messageType=sensor_msgs/LaserScan  SampleTime=-1  legacyBusStruct=off  messageQueueLength=1
  Subscribe1 : robotlib/Subscribe  topicSource=Select from ROS network  topic=/robot3/odom  messageType=nav_msgs/Odometry  SampleTime=-1  legacyBusStruct=off  messageQueueLength=1
  Terminator : Terminator
  Waypoints Input1 : Constant  Value=Way3  OutDataTypeStr=double
  quad2eul : MATLAB Function  TreatAsAtomicUnit=on
  NewMessage : Outport
  LIDAR : Outport  Port=2
  POSE : Outport  Port=3
  Waypoints : Outport  Port=4
  wires:
  Bus Selector/6 -> quad2eul/4(W)  "<W>"
  Bus Selector/1 -> Mux/1  "<X>"
  quad2eul/1(Yaw) -> Mux/3
  Bus Selector/4 -> quad2eul/2(Y)  "<Y>"
  Subscribe1/2 -> Bus Selector/1
  MATLAB Function/1(Ranges) -> Mux1/1
  Mux/1 -> POSE/1
  Subscribe/2 -> MATLAB Function/1(LaserScanMsg)
  Subscribe/1 -> NewMessage/1
  Subscribe1/1 -> Terminator/1
  Bus Selector/3 -> quad2eul/1(X)  "<X>"
  Bus Selector/2 -> Mux/2  "<Y>"
  MATLAB Function/2(Angles) -> Mux1/2
  Mux1/1 -> LIDAR/1
  Waypoints Input1/1 -> Waypoints/1
  Bus Selector/5 -> quad2eul/3(Z)  "<Z>"

== system Four_Robots_v2/TurtleBot3/Outputs ==
  NewMessage : Inport
  dV : Inport  Port=2
  dW : Inport  Port=3
  V : Inport  Port=4
  W : Inport  Port=5
  CloseToGoal : Inport  Port=6
  LIDAR : Inport  Port=7
  POSE : Inport  Port=8
  TargetDir : Inport  Port=9
  DVelocities : Scope  NumInputPorts=2
  Outputs : Subsystem
  wires:
  POSE/1 -> Outputs/7(POSE)
  V/1 -> Outputs/3(V)
  NewMessage/1 -> Outputs/Enable
  CloseToGoal/1 -> Outputs/5(CloseToGoal)
  LIDAR/1 -> Outputs/6(LIDAR)
  TargetDir/1 -> Outputs/8(TargetDir)
  W/1 -> Outputs/4(W)
  dV/1 -> DVelocities/1, Outputs/1(dV)
  dW/1 -> DVelocities/2, Outputs/2(dW)

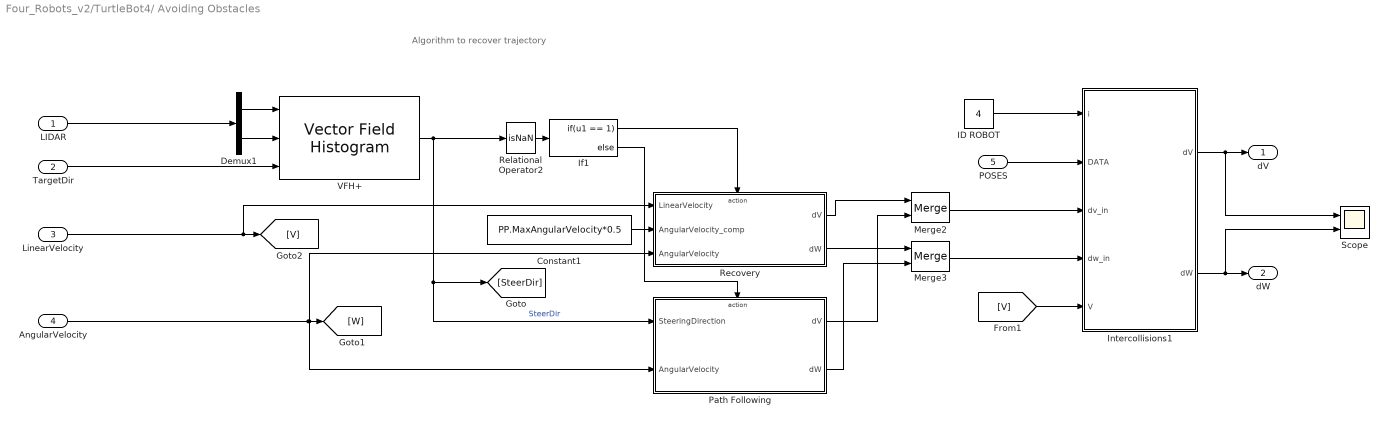
== system Four_Robots_v2/TurtleBot4/ Avoiding Obstacles ==
  note: Algorithm to recover trajectory
  LIDAR : Inport
  TargetDir : Inport  Port=2
  LinearVelocity : Inport  Port=3
  AngularVelocity : Inport  Port=4
  POSES : Inport  Port=5
  Constant1 : Constant  Value=PP.MaxAngularVelocity*0.5
  Demux1 : Demux  Outputs=2
  ID ROBOT : Constant  Value=4
  If1 : If  IfExpression=u1 == 1
  Intercollisions1 : MATLAB Function  TreatAsAtomicUnit=on
  Merge2 : Merge
  Merge3 : Merge
  Path Following : Subsystem  TreatAsAtomicUnit=on
  Recovery : Subsystem  TreatAsAtomicUnit=on
  Relational Operator2 : RelationalOperator  Operator=isNaN  OutDataTypeStr=boolean  RndMeth=Simplest
  Scope : Scope  NumInputPorts=2
  VFH+ : robotalgslib/Vector Field Histogram  NumAngularSectors=VFH.NumAngularSectors  DistanceLimits=VFH.DistanceLimits  HistogramThresholds=VFH.HistogramThresholds  RobotRadius=VFH.RobotRadius  SafetyDistance=VFH.SafetyDistance  MinTurningRadius=VFH.MinTurningRadius  SimulateUsing=Code generation  TargetDirectionWeight=5  CurrentDirectionWeight=2  PreviousDirectionWeight=2
      settings: SourceProductBaseCode=NV,RO
  dV : Outport
  dW : Outport  Port=2
  wires:
  ID ROBOT/1 -> Intercollisions1/1(i)
  POSES/1 -> Intercollisions1/2(DATA)
  Intercollisions1/1(dV) -> dV/1, Scope/1
  Intercollisions1/2(dW) -> dW/1, Scope/2
  Merge2/1 -> Intercollisions1/3(dv_in)
  [V] -> Intercollisions1/5(V)
  Merge3/1 -> Intercollisions1/4(dw_in)
  Demux1/2 -> VFH+/2
  If1/2 -> Path Following/Action
  Path Following/1(dV) -> Merge2/2
  Path Following/2(dW) -> Merge3/2
  VFH+/1 -> Relational Operator2/1, Path Following/1(SteeringDirection), [SteerDir]  "SteerDir"
  LIDAR/1 -> Demux1/1
  LinearVelocity/1 -> Recovery/1(LinearVelocity), [V]
  Relational Operator2/1 -> If1/1
  TargetDir/1 -> VFH+/3
  Demux1/1 -> VFH+/1
  AngularVelocity/1 -> [W], Path Following/2(AngularVelocity), Recovery/3(AngularVelocity)
  Recovery/2(dW) -> Merge3/1
  Recovery/1(dV) -> Merge2/1
  Constant1/1 -> Recovery/2(AngularVelocity_comp)
  If1/1 -> Recovery/Action

== system Four_Robots_v2/TurtleBot4/ Path following ==
  note: Check If Close To Goal
  POSE : Inport
  Waypoints : Inport  Port=2
  " Extract Goal" : MATLAB Function  TreatAsAtomicUnit=on
  Dot Product : DotProduct  InputSameDT=on  OutDataTypeStr=Inherit: Inherit via internal rule
  GoalRadius : Constant  Value=0.15
  Pure Pursuit : robotalgslib/Pure Pursuit  DesiredLinearVelocity=PP.DesiredLinearVelocity  MaxAngularVelocity=PP.MaxAngularVelocity  LookaheadDistance=PP.LookaheadDistance  TargetDirPort=on  SimulateUsing=Code generation
  Relational Operator : RelationalOperator  Operator=<=  OutDataTypeStr=boolean  RndMeth=Simplest
  Selector : Selector  InputPortWidth=3  IndexOptions=Index vector (dialog)  Indices=[1 2]  OutputSizes=1
  Sqrt : Sqrt  SaturateOnIntegerOverflow=on
  Subtract : Sum  Inputs=|+-
  TargetDir : Outport
  LinVel : Outport  Port=2
  AngVel : Outport  Port=3
  ClosetoGoal : Outport  Port=4
  wires:
  POSE/1 -> Pure Pursuit/1, Selector/1
  GoalRadius/1 -> Relational Operator/2
  Sqrt/1 -> Relational Operator/1
  Waypoints/1 -> Pure Pursuit/2, " Extract Goal"/1(Waypoints)
  Selector/1 -> Subtract/1
  Pure Pursuit/1 -> LinVel/1
  Dot Product/1 -> Sqrt/1
  " Extract Goal"/1(Goal) -> Subtract/2
  Subtract/1 -> Dot Product/2, Dot Product/1
  Relational Operator/1 -> ClosetoGoal/1
  Pure Pursuit/2 -> AngVel/1
  Pure Pursuit/3 -> TargetDir/1

== system Four_Robots_v2/TurtleBot4/Inputs ==
  note: Receive Robot Pose
  note: Receive Laser Message
  Bus Selector : BusSelector  OutputSignals=Pose.Pose.Position.X,Pose.Pose.Position.Y,Pose.Pose.Orientation.X,Pose.Pose.Orientation.Y,Pose.Pose.Orientation.Z,Pose.Pose.Orientation.W
  MATLAB Function : MATLAB Function  TreatAsAtomicUnit=on
  Mux : Mux  Inputs=3
  Mux1 : Mux  Inputs=2
  Subscribe : robotlib/Subscribe  topicSource=Select from ROS network  topic=/robot4/scan  messageType=sensor_msgs/LaserScan  SampleTime=-1  legacyBusStruct=off  messageQueueLength=1
  Subscribe1 : robotlib/Subscribe  topicSource=Select from ROS network  topic=/robot4/odom  messageType=nav_msgs/Odometry  SampleTime=-1  legacyBusStruct=off  messageQueueLength=1
  Terminator : Terminator
  Waypoints Input1 : Constant  Value=Way4  OutDataTypeStr=double
  quad2eul : MATLAB Function  TreatAsAtomicUnit=on
  NewMessage : Outport
  LIDAR : Outport  Port=2
  POSE : Outport  Port=3
  Waypoints : Outport  Port=4
  wires:
  Bus Selector/5 -> quad2eul/3(Z)  "<Z>"
  Waypoints Input1/1 -> Waypoints/1
  Mux1/1 -> LIDAR/1
  MATLAB Function/2(Angles) -> Mux1/2
  Bus Selector/2 -> Mux/2  "<Y>"
  Bus Selector/3 -> quad2eul/1(X)  "<X>"
  Subscribe1/1 -> Terminator/1
  Subscribe/1 -> NewMessage/1
  Subscribe/2 -> MATLAB Function/1(LaserScanMsg)
  Mux/1 -> POSE/1
  MATLAB Function/1(Ranges) -> Mux1/1
  Subscribe1/2 -> Bus Selector/1
  Bus Selector/4 -> quad2eul/2(Y)  "<Y>"
  quad2eul/1(Yaw) -> Mux/3
  Bus Selector/1 -> Mux/1  "<X>"
  Bus Selector/6 -> quad2eul/4(W)  "<W>"

== system Four_Robots_v2/TurtleBot4/Outputs ==
  NewMessage : Inport
  dV : Inport  Port=2
  dW : Inport  Port=3
  V : Inport  Port=4
  W : Inport  Port=5
  CloseToGoal : Inport  Port=6
  LIDAR : Inport  Port=7
  POSE : Inport  Port=8
  TargetDir : Inport  Port=9
  DVelocities : Scope  NumInputPorts=2
  Outputs : Subsystem
  wires:
  dW/1 -> Outputs/2(dW), DVelocities/2
  dV/1 -> Outputs/1(dV), DVelocities/1
  W/1 -> Outputs/4(W)
  TargetDir/1 -> Outputs/8(TargetDir)
  LIDAR/1 -> Outputs/6(LIDAR)
  CloseToGoal/1 -> Outputs/5(CloseToGoal)
  NewMessage/1 -> Outputs/Enable
  V/1 -> Outputs/3(V)
  POSE/1 -> Outputs/7(POSE)

== system Four_Robots_v2/TurtleBot1/ Avoiding Obstacles/Path Following ==
  SteeringDirection : Inport
  AngularVelocity : Inport  Port=2
  Action Port : ActionPort  ActionPortLabel=else
  Compute Angular Velocity : MATLAB Function  TreatAsAtomicUnit=on
  Constant : Constant  Value=0
  MaxAngularVelocity : Constant  Value=1.82
  Subtract : Sum  Inputs=+-
  dV : Outport  VectorParamsAs1DForOutWhenUnconnected=off
  dW : Outport  Port=2  VectorParamsAs1DForOutWhenUnconnected=off
  wires:
  AngularVelocity/1 -> Subtract/2
  Compute Angular Velocity/1(w) -> Subtract/1
  Subtract/1 -> dW/1
  SteeringDirection/1 -> Compute Angular Velocity/1(steeringDir)
  MaxAngularVelocity/1 -> Compute Angular Velocity/2(wMax)
  Constant/1 -> dV/1

== system Four_Robots_v2/TurtleBot1/ Avoiding Obstacles/Recovery ==
  LinearVelocity : Inport
  AngularVelocity_comp : Inport  Port=2
  AngularVelocity : Inport  Port=3
  Action Port : ActionPort  ActionPortLabel=if(u1 == 1)
  Gain : Gain  Gain=-1
  Subtract : Sum  Inputs=|+-
  dV : Outport  VectorParamsAs1DForOutWhenUnconnected=off
  dW : Outport  Port=2  VectorParamsAs1DForOutWhenUnconnected=off
  wires:
  Subtract/1 -> dW/1
  AngularVelocity/1 -> Subtract/2
  Gain/1 -> dV/1
  LinearVelocity/1 -> Gain/1
  AngularVelocity_comp/1 -> Subtract/1

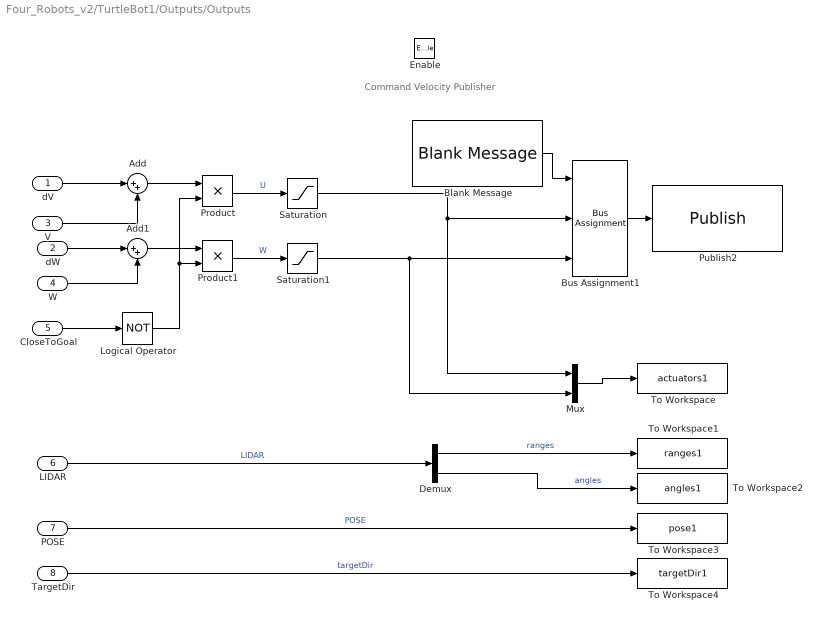
== system Four_Robots_v2/TurtleBot1/Outputs/Outputs ==
  note: Command Velocity Publisher
  dV : Inport
  dW : Inport  Port=2
  V : Inport  Port=3
  W : Inport  Port=4
  CloseToGoal : Inport  Port=5
  LIDAR : Inport  Port=6
  POSE : Inport  Port=7
  TargetDir : Inport  Port=8
  Enable : EnablePort
  Add : Sum  Inputs=|++
  Add1 : Sum  Inputs=|++
  Blank Message : robotlib/Blank Message  messageClass=Message  entityType=geometry_msgs/Twist  messageType=geometry_msgs/Twist  SampleTime=inf  legacyBusStruct=off
  Bus Assignment1 : BusAssignment  DialogController=Simulink.DDGSource_BusAssignment  AssignedSignals=Linear.X,Angular.Z
  Demux : Demux  Outputs=2
  Logical Operator : Logic  Operator=NOT  AllPortsSameDT=off  OutDataTypeStr=boolean
  Mux : Mux  Inputs=2
  Product : Product
  Product1 : Product
  Publish2 : robotlib/Publish  topicSource=Select from ROS network  topic=/robot1/cmd_vel  messageType=geometry_msgs/Twist  legacyBusStruct=off  messageQueueLength=105
  Saturation : Saturate  UpperLimit=PP.DesiredLinearVelocity  LowerLimit=-PP.DesiredLinearVelocity
  Saturation1 : Saturate  UpperLimit=PP.MaxAngularVelocity  LowerLimit=-PP.MaxAngularVelocity
  To Workspace : ToWorkspace  VariableName=actuators1  SaveFormat=Structure With Time  SampleTime=0.01
      settings: Decimation=2
  To Workspace1 : ToWorkspace  VariableName=ranges1  SaveFormat=Structure With Time  SampleTime=0.01
      settings: Decimation=2
  To Workspace2 : ToWorkspace  VariableName=angles1  SaveFormat=Structure With Time  SampleTime=0.01
      settings: Decimation=2
  To Workspace3 : ToWorkspace  VariableName=pose1  SaveFormat=Structure With Time  SampleTime=0.01
      settings: Decimation=2
  To Workspace4 : ToWorkspace  VariableName=targetDir1  SaveFormat=Structure With Time  SampleTime=0.01
      settings: Decimation=2
  wires:
  V/1 -> Add/2
  W/1 -> Add1/2
  dV/1 -> Add/1
  dW/1 -> Add1/1
  CloseToGoal/1 -> Logical Operator/1
  Add/1 -> Product/1
  Add1/1 -> Product1/1
  Blank Message/1 -> Bus Assignment1/1
  Bus Assignment1/1 -> Publish2/1
  Logical Operator/1 -> Product1/2, Product/2
  Mux/1 -> To Workspace/1
  Product/1 -> Saturation/1  "U"
  Saturation/1 -> Mux/1, Bus Assignment1/2
  Product1/1 -> Saturation1/1  "W"
  Saturation1/1 -> Mux/2, Bus Assignment1/3
  TargetDir/1 -> To Workspace4/1  "targetDir"
  Demux/2 -> To Workspace2/1  "angles"
  LIDAR/1 -> Demux/1  "LIDAR"
  POSE/1 -> To Workspace3/1  "POSE"
  Demux/1 -> To Workspace1/1  "ranges"

== system Four_Robots_v2/TurtleBot2/ Avoiding Obstacles/Path Following ==
  SteeringDirection : Inport
  AngularVelocity : Inport  Port=2
  Action Port : ActionPort  ActionPortLabel=else
  Compute Angular Velocity : MATLAB Function  TreatAsAtomicUnit=on
  Constant : Constant  Value=0
  MaxAngularVelocity : Constant  Value=1.82
  Subtract : Sum  Inputs=+-
  dV : Outport  VectorParamsAs1DForOutWhenUnconnected=off
  dW : Outport  Port=2  VectorParamsAs1DForOutWhenUnconnected=off
  wires:
  AngularVelocity/1 -> Subtract/2
  Compute Angular Velocity/1(w) -> Subtract/1
  Subtract/1 -> dW/1
  SteeringDirection/1 -> Compute Angular Velocity/1(steeringDir)
  MaxAngularVelocity/1 -> Compute Angular Velocity/2(wMax)
  Constant/1 -> dV/1

== system Four_Robots_v2/TurtleBot2/ Avoiding Obstacles/Recovery ==
  LinearVelocity : Inport
  AngularVelocity_comp : Inport  Port=2
  AngularVelocity : Inport  Port=3
  Action Port : ActionPort  ActionPortLabel=if(u1 == 1)
  Gain : Gain  Gain=-1
  Subtract : Sum  Inputs=|+-
  dV : Outport  VectorParamsAs1DForOutWhenUnconnected=off
  dW : Outport  Port=2  VectorParamsAs1DForOutWhenUnconnected=off
  wires:
  Subtract/1 -> dW/1
  AngularVelocity/1 -> Subtract/2
  Gain/1 -> dV/1
  LinearVelocity/1 -> Gain/1
  AngularVelocity_comp/1 -> Subtract/1

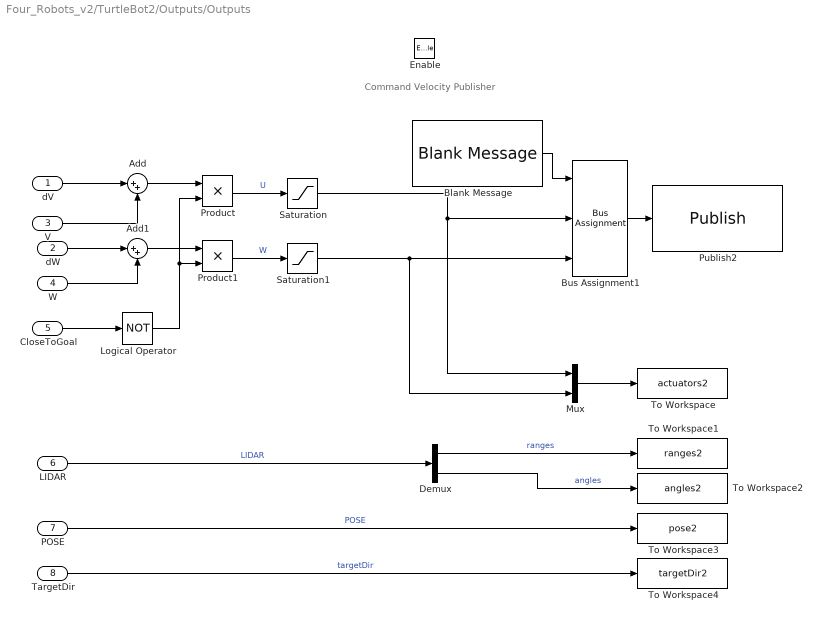
== system Four_Robots_v2/TurtleBot2/Outputs/Outputs ==
  note: Command Velocity Publisher
  dV : Inport
  dW : Inport  Port=2
  V : Inport  Port=3
  W : Inport  Port=4
  CloseToGoal : Inport  Port=5
  LIDAR : Inport  Port=6
  POSE : Inport  Port=7
  TargetDir : Inport  Port=8
  Enable : EnablePort
  Add : Sum  Inputs=|++
  Add1 : Sum  Inputs=|++
  Blank Message : robotlib/Blank Message  messageClass=Message  entityType=geometry_msgs/Twist  messageType=geometry_msgs/Twist  SampleTime=inf  legacyBusStruct=off
  Bus Assignment1 : BusAssignment  DialogController=Simulink.DDGSource_BusAssignment  AssignedSignals=Linear.X,Angular.Z
  Demux : Demux  Outputs=2
  Logical Operator : Logic  Operator=NOT  AllPortsSameDT=off  OutDataTypeStr=boolean
  Mux : Mux  Inputs=2
  Product : Product
  Product1 : Product
  Publish2 : robotlib/Publish  topicSource=Select from ROS network  topic=/robot2/cmd_vel  messageType=geometry_msgs/Twist  legacyBusStruct=off  messageQueueLength=105
  Saturation : Saturate  UpperLimit=PP.DesiredLinearVelocity  LowerLimit=-PP.DesiredLinearVelocity
  Saturation1 : Saturate  UpperLimit=PP.MaxAngularVelocity  LowerLimit=-PP.MaxAngularVelocity
  To Workspace : ToWorkspace  VariableName=actuators2  SaveFormat=Structure With Time  SampleTime=0.01
      settings: Decimation=2
  To Workspace1 : ToWorkspace  VariableName=ranges2  SaveFormat=Structure With Time  SampleTime=0.01
      settings: Decimation=2
  To Workspace2 : ToWorkspace  VariableName=angles2  SaveFormat=Structure With Time  SampleTime=0.01
      settings: Decimation=2
  To Workspace3 : ToWorkspace  VariableName=pose2  SaveFormat=Structure With Time  SampleTime=0.01
      settings: Decimation=2
  To Workspace4 : ToWorkspace  VariableName=targetDir2  SaveFormat=Structure With Time  SampleTime=0.01
      settings: Decimation=2
  wires:
  V/1 -> Add/2
  W/1 -> Add1/2
  dV/1 -> Add/1
  dW/1 -> Add1/1
  CloseToGoal/1 -> Logical Operator/1
  Add/1 -> Product/1
  Add1/1 -> Product1/1
  Blank Message/1 -> Bus Assignment1/1
  Bus Assignment1/1 -> Publish2/1
  Logical Operator/1 -> Product1/2, Product/2
  Mux/1 -> To Workspace/1
  Product/1 -> Saturation/1  "U"
  Saturation/1 -> Mux/1, Bus Assignment1/2
  Product1/1 -> Saturation1/1  "W"
  Saturation1/1 -> Mux/2, Bus Assignment1/3
  TargetDir/1 -> To Workspace4/1  "targetDir"
  Demux/2 -> To Workspace2/1  "angles"
  LIDAR/1 -> Demux/1  "LIDAR"
  POSE/1 -> To Workspace3/1  "POSE"
  Demux/1 -> To Workspace1/1  "ranges"

== system Four_Robots_v2/TurtleBot3/ Avoiding Obstacles/Path Following ==
  SteeringDirection : Inport
  AngularVelocity : Inport  Port=2
  Action Port : ActionPort  ActionPortLabel=else
  Compute Angular Velocity : MATLAB Function  TreatAsAtomicUnit=on
  Constant : Constant  Value=0
  MaxAngularVelocity : Constant  Value=1.82
  Subtract : Sum  Inputs=+-
  dV : Outport  VectorParamsAs1DForOutWhenUnconnected=off
  dW : Outport  Port=2  VectorParamsAs1DForOutWhenUnconnected=off
  wires:
  AngularVelocity/1 -> Subtract/2
  Compute Angular Velocity/1(w) -> Subtract/1
  Subtract/1 -> dW/1
  SteeringDirection/1 -> Compute Angular Velocity/1(steeringDir)
  MaxAngularVelocity/1 -> Compute Angular Velocity/2(wMax)
  Constant/1 -> dV/1

== system Four_Robots_v2/TurtleBot3/ Avoiding Obstacles/Recovery ==
  LinearVelocity : Inport
  AngularVelocity_comp : Inport  Port=2
  AngularVelocity : Inport  Port=3
  Action Port : ActionPort  ActionPortLabel=if(u1 == 1)
  Gain : Gain  Gain=-1
  Subtract : Sum  Inputs=|+-
  dV : Outport  VectorParamsAs1DForOutWhenUnconnected=off
  dW : Outport  Port=2  VectorParamsAs1DForOutWhenUnconnected=off
  wires:
  Subtract/1 -> dW/1
  AngularVelocity/1 -> Subtract/2
  Gain/1 -> dV/1
  LinearVelocity/1 -> Gain/1
  AngularVelocity_comp/1 -> Subtract/1

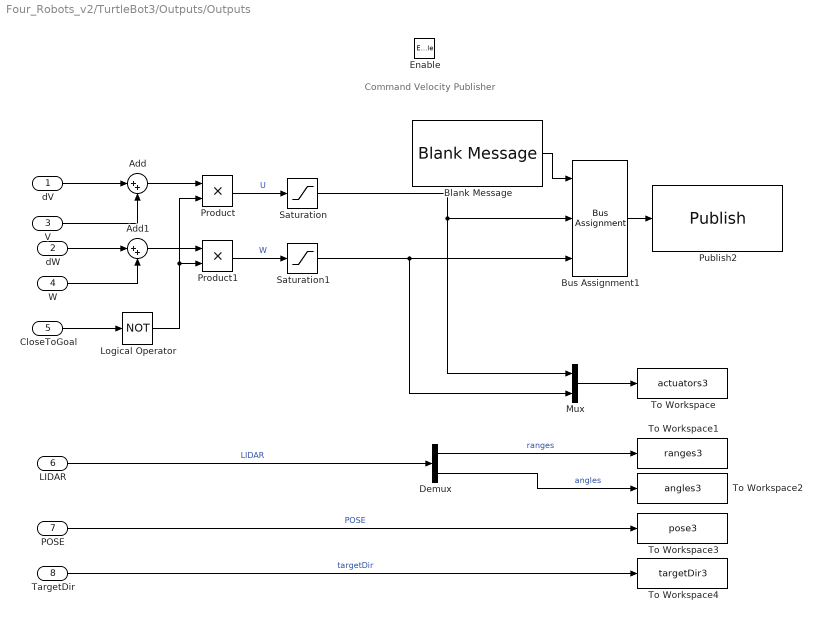
== system Four_Robots_v2/TurtleBot3/Outputs/Outputs ==
  note: Command Velocity Publisher
  dV : Inport
  dW : Inport  Port=2
  V : Inport  Port=3
  W : Inport  Port=4
  CloseToGoal : Inport  Port=5
  LIDAR : Inport  Port=6
  POSE : Inport  Port=7
  TargetDir : Inport  Port=8
  Enable : EnablePort
  Add : Sum  Inputs=|++
  Add1 : Sum  Inputs=|++
  Blank Message : robotlib/Blank Message  messageClass=Message  entityType=geometry_msgs/Twist  messageType=geometry_msgs/Twist  SampleTime=inf  legacyBusStruct=off
  Bus Assignment1 : BusAssignment  DialogController=Simulink.DDGSource_BusAssignment  AssignedSignals=Linear.X,Angular.Z
  Demux : Demux  Outputs=2
  Logical Operator : Logic  Operator=NOT  AllPortsSameDT=off  OutDataTypeStr=boolean
  Mux : Mux  Inputs=2
  Product : Product
  Product1 : Product
  Publish2 : robotlib/Publish  topicSource=Select from ROS network  topic=/robot3/cmd_vel  messageType=geometry_msgs/Twist  legacyBusStruct=off  messageQueueLength=105
  Saturation : Saturate  UpperLimit=PP.DesiredLinearVelocity  LowerLimit=-PP.DesiredLinearVelocity
  Saturation1 : Saturate  UpperLimit=PP.MaxAngularVelocity  LowerLimit=-PP.MaxAngularVelocity
  To Workspace : ToWorkspace  VariableName=actuators3  SaveFormat=Structure With Time  SampleTime=0.01
      settings: Decimation=2
  To Workspace1 : ToWorkspace  VariableName=ranges3  SaveFormat=Structure With Time  SampleTime=0.01
      settings: Decimation=2
  To Workspace2 : ToWorkspace  VariableName=angles3  SaveFormat=Structure With Time  SampleTime=0.01
      settings: Decimation=2
  To Workspace3 : ToWorkspace  VariableName=pose3  SaveFormat=Structure With Time  SampleTime=0.01
      settings: Decimation=2
  To Workspace4 : ToWorkspace  VariableName=targetDir3  SaveFormat=Structure With Time  SampleTime=0.01
      settings: Decimation=2
  wires:
  V/1 -> Add/2
  W/1 -> Add1/2
  dV/1 -> Add/1
  dW/1 -> Add1/1
  CloseToGoal/1 -> Logical Operator/1
  Add/1 -> Product/1
  Add1/1 -> Product1/1
  Blank Message/1 -> Bus Assignment1/1
  Bus Assignment1/1 -> Publish2/1
  Logical Operator/1 -> Product1/2, Product/2
  Mux/1 -> To Workspace/1
  Product/1 -> Saturation/1  "U"
  Saturation/1 -> Mux/1, Bus Assignment1/2
  Product1/1 -> Saturation1/1  "W"
  Saturation1/1 -> Mux/2, Bus Assignment1/3
  TargetDir/1 -> To Workspace4/1  "targetDir"
  Demux/2 -> To Workspace2/1  "angles"
  LIDAR/1 -> Demux/1  "LIDAR"
  POSE/1 -> To Workspace3/1  "POSE"
  Demux/1 -> To Workspace1/1  "ranges"
